simulink model "kinovaMicoSimscapeModel"  (R2021b)
(part 42 of 50)

Y6_20_4=(3*dq2*dqr3*sin(2*q6))/128 + (3*dq3*dqr2*sin(2*q6))/128 - (3*dq3*dqr3*sin(2*q6))/128 + (3*dq2*dqr3*cos(2*q6)*sin(q5))/16 + (3*dq2*dqr3*sin(2*q6)*cos(q5))/32 - (3*dq3*dqr3*cos(2*q6)*sin(q5))/16 - (3*dq3*dqr3*sin(2*q6)*cos(q5))/32 + (3^(1/2)*dq4*dqr3*sin(q4))/8 + (27*dq2*dqr3*cos(2*q4)*sin(2*q6))/128 + (27*dq3*dqr2*cos(2*q4)*sin(2*q6))/128 - (15*dq2*dqr3*cos(2*q5)*sin(2*q6))/128 - (3*dq2*dqr3*cos(2*q6)*sin(2*q5))/32 - (15*dq3*dqr2*cos(2*q5)*sin(2*q6))/128 - (27*dq3*dqr3*cos(2*q4)*sin(2*q6))/128 + (15*dq3*dqr3*cos(2*q5)*sin(2*q6))/128 + (3*dq3*dqr3*cos(2*q6)*sin(2*q5))/32 - (dq1*dqr3*cos(q2)*sin(q3))/8 + (dq1*dqr3*cos(q3)*sin(q2))/8 - (3^(1/2)*dq4*dqr3*cos(q4)*sin(q5))/4 - (3^(1/2)*dq4*dqr3*cos(q5)*sin(q4))/8 - (3^(1/2)*dq5*dqr3*cos(q4)*sin(q5))/8 - (3^(1/2)*dq5*dqr3*cos(q5)*sin(q4))/4 + (3*dq2*dqr3*cos(2*q4)*cos(2*q6)*sin(q5))/16 + (3*dq2*dqr3*cos(2*q4)*sin(2*q6)*cos(q5))/32 + (3*dq2*dqr3*cos(2*q6)*sin(2*q4)*cos(q5))/8 - (3*dq3*dqr3*cos(2*q4)*cos(2*q6)*sin(q5))/16 - (3*dq3*dqr3*cos(2*q4)*sin(2*q6)*cos(q5))/32 - (3*dq3*dqr3*cos(2*q6)*sin(2*q4)*cos(q5))/8 - (3*dq2*dqr3*sin(2*q4)*sin(2*q6)*sin(q5))/16 + (3*dq3*dqr3*sin(2*q4)*sin(2*q6)*sin(q5))/16 + (9*3^(1/2)*dq4*dqr3*sin(2*q6)*cos(q4))/64 + (3*3^(1/2)*dq5*dqr3*sin(2*q6)*cos(q4))/16 - (3*dq1*dqr3*cos(q2)*cos(q5)*sin(q3))/8 + (3*dq1*dqr3*cos(q3)*cos(q5)*sin(q2))/8 + (25*dq2*dqr3*cos(2*q4)*cos(2*q5)*sin(2*q6))/128 + (5*dq2*dqr3*cos(2*q4)*cos(2*q6)*sin(2*q5))/32 + (dq2*dqr3*cos(2*q5)*cos(2*q6)*sin(2*q4))/8 + (25*dq3*dqr2*cos(2*q4)*cos(2*q5)*sin(2*q6))/128 - (25*dq3*dqr3*cos(2*q4)*cos(2*q5)*sin(2*q6))/128 - (5*dq3*dqr3*cos(2*q4)*cos(2*q6)*sin(2*q5))/32 - (dq3*dqr3*cos(2*q5)*cos(2*q6)*sin(2*q4))/8 - (5*dq2*dqr3*sin(2*q4)*sin(2*q5)*sin(2*q6))/32 + (5*dq3*dqr3*sin(2*q4)*sin(2*q5)*sin(2*q6))/32 + (3*dq1*dqr4*cos(2*q6)*sin(q2)*sin(q3)*sin(q5))/8 + (3*dq1*dqr4*sin(2*q6)*cos(q5)*sin(q2)*sin(q3))/16 - (3^(1/2)*dq1*dqr3*cos(q2)*cos(q3)*sin(q4))/8 - (3^(1/2)*dq1*dqr3*sin(q2)*sin(q3)*sin(q4))/8 - (27*dq1*dqr3*sin(2*q4)*sin(2*q6)*cos(q2)*sin(q3))/128 + (27*dq1*dqr3*sin(2*q4)*sin(2*q6)*cos(q3)*sin(q2))/128 - (3*dq1*dqr4*cos(2*q6)*sin(2*q5)*sin(q2)*sin(q3))/16 - (3^(1/2)*dq4*dqr3*cos(2*q6)*cos(q4)*sin(q5))/8 + (3^(1/2)*dq4*dqr3*cos(2*q6)*cos(q5)*sin(q4))/8 - (3^(1/2)*dq4*dqr3*sin(2*q6)*cos(q4)*cos(q5))/16 + (3^(1/2)*dq5*dqr3*cos(2*q6)*cos(q4)*sin(q5))/8 + (3^(1/2)*dq5*dqr3*cos(2*q6)*cos(q5)*sin(q4))/4 + (3^(1/2)*dq5*dqr3*sin(2*q6)*cos(q4)*cos(q5))/16 - (3^(1/2)*dq4*dqr3*sin(2*q6)*sin(q4)*sin(q5))/16 - (3^(1/2)*dq5*dqr3*sin(2*q6)*sin(q4)*sin(q5))/8 - (3^(1/2)*dq4*dqr3*cos(2*q5)*cos(2*q6)*sin(q4))/8 - (5*3^(1/2)*dq4*dqr3*cos(2*q5)*sin(2*q6)*cos(q4))/64 - (3^(1/2)*dq4*dqr3*cos(2*q6)*sin(2*q5)*cos(q4))/16 + (5*3^(1/2)*dq4*dqr3*sin(2*q5)*sin(2*q6)*sin(q4))/32 + (3^(1/2)*dq1*dqr3*cos(q4)*sin(q2)*sin(q3)*sin(q5))/4 + (3^(1/2)*dq1*dqr3*cos(q5)*sin(q2)*sin(q3)*sin(q4))/8 + (3*dq1*dqr3*cos(2*q4)*cos(2*q6)*cos(q2)*cos(q5)*sin(q3))/8 - (3*dq1*dqr3*cos(2*q4)*cos(2*q6)*cos(q3)*cos(q5)*sin(q2))/8 - (3*dq1*dqr3*cos(2*q4)*sin(2*q6)*cos(q2)*sin(q3)*sin(q5))/16 + (3*dq1*dqr3*cos(2*q4)*sin(2*q6)*cos(q3)*sin(q2)*sin(q5))/16 - (3*dq1*dqr3*cos(2*q6)*sin(2*q4)*cos(q2)*sin(q3)*sin(q5))/16 + (3*dq1*dqr3*cos(2*q6)*sin(2*q4)*cos(q3)*sin(q2)*sin(q5))/16 - (3*dq1*dqr3*sin(2*q4)*sin(2*q6)*cos(q2)*cos(q5)*sin(q3))/32 + (3*dq1*dqr3*sin(2*q4)*sin(2*q6)*cos(q3)*cos(q5)*sin(q2))/32 + (9*3^(1/2)*dq1*dqr3*sin(2*q6)*cos(q2)*cos(q3)*cos(q4))/64 + (9*3^(1/2)*dq1*dqr3*sin(2*q6)*cos(q4)*sin(q2)*sin(q3))/64 + (dq1*dqr3*cos(2*q4)*cos(2*q5)*cos(2*q6)*cos(q2)*sin(q3))/8 - (dq1*dqr3*cos(2*q4)*cos(2*q5)*cos(2*q6)*cos(q3)*sin(q2))/8 - (5*dq1*dqr3*cos(2*q4)*sin(2*q5)*sin(2*q6)*cos(q2)*sin(q3))/32 + (5*dq1*dqr3*cos(2*q4)*sin(2*q5)*sin(2*q6)*cos(q3)*sin(q2))/32 - (25*dq1*dqr3*cos(2*q5)*sin(2*q4)*sin(2*q6)*cos(q2)*sin(q3))/128 + (25*dq1*dqr3*cos(2*q5)*sin(2*q4)*sin(2*q6)*cos(q3)*sin(q2))/128 - (5*dq1*dqr3*cos(2*q6)*sin(2*q4)*sin(2*q5)*cos(q2)*sin(q3))/32 + (5*dq1*dqr3*cos(2*q6)*sin(2*q4)*sin(2*q5)*cos(q3)*sin(q2))/32 + (3^(1/2)*dq1*dqr3*cos(q2)*cos(q3)*cos(q4)*sin(q5))/4 + (3^(1/2)*dq1*dqr3*cos(q2)*cos(q3)*cos(q5)*sin(q4))/8 - (3^(1/2)*dq1*dqr3*cos(2*q6)*cos(q2)*cos(q3)*cos(q4)*sin(q5))/8 + (3^(1/2)*dq1*dqr3*cos(2*q6)*cos(q2)*cos(q3)*cos(q5)*sin(q4))/8 - (3^(1/2)*dq1*dqr3*sin(2*q6)*cos(q2)*cos(q3)*cos(q4)*cos(q5))/16 - (3^(1/2)*dq1*dqr3*cos(2*q6)*cos(q4)*sin(q2)*sin(q3)*sin(q5))/8 + (3^(1/2)*dq1*dqr3*cos(2*q6)*cos(q5)*sin(q2)*sin(q3)*sin(q4))/8 - (3^(1/2)*dq1*dqr3*sin(2*q6)*cos(q2)*cos(q3)*sin(q4)*sin(q5))/16 - (3^(1/2)*dq1*dqr3*sin(2*q6)*cos(q4)*cos(q5)*sin(q2)*sin(q3))/16 - (3^(1/2)*dq1*dqr3*sin(2*q6)*sin(q2)*sin(q3)*sin(q4)*sin(q5))/16 - (3^(1/2)*dq1*dqr3*cos(2*q5)*cos(2*q6)*cos(q2)*cos(q3)*sin(q4))/8 - (5*3^(1/2)*dq1*dqr3*cos(2*q5)*sin(2*q6)*cos(q2)*cos(q3)*cos(q4))/64 - (3^(1/2)*dq1*dqr3*cos(2*q6)*sin(2*q5)*cos(q2)*cos(q3)*cos(q4))/16 - (3^(1/2)*dq1*dqr3*cos(2*q5)*cos(2*q6)*sin(q2)*sin(q3)*sin(q4))/8 - (5*3^(1/2)*dq1*dqr3*cos(2*q5)*sin(2*q6)*cos(q4)*sin(q2)*sin(q3))/64 - (3^(1/2)*dq1*dqr3*cos(2*q6)*sin(2*q5)*cos(q4)*sin(q2)*sin(q3))/16 + (5*3^(1/2)*dq1*dqr3*sin(2*q5)*sin(2*q6)*cos(q2)*cos(q3)*sin(q4))/32 + (5*3^(1/2)*dq1*dqr3*sin(2*q5)*sin(2*q6)*sin(q2)*sin(q3)*sin(q4))/32;
Y6_20_5=(3*dq4*dqr4*sin(2*q6))/64 - (3*dq5*dqr4*sin(q5))/8 - (3*dq4*dqr5*sin(q5))/8 - (3*dq5*dqr4*sin(2*q6))/16 + (3*dq4*dqr4*cos(2*q6)*sin(q5))/8 + (3*dq4*dqr4*sin(2*q6)*cos(q5))/16 + (3*dq4*dqr5*cos(2*q6)*sin(q5))/8 + (3*dq5*dqr4*cos(2*q6)*sin(q5))/8 + (3*dq5*dqr4*sin(2*q6)*cos(q5))/16 - (3^(1/2)*dq2*dqr4*sin(q4))/8 + (3^(1/2)*dq3*dqr4*sin(q4))/8 - (15*dq4*dqr4*cos(2*q5)*sin(2*q6))/64 - (3*dq4*dqr4*cos(2*q6)*sin(2*q5))/16 + (3*dq1*dqr4*sin(2*q6)*cos(q2)*cos(q3))/64 - (3*dq1*dqr5*sin(2*q6)*cos(q2)*cos(q3))/16 + (3*dq1*dqr4*sin(2*q6)*sin(q2)*sin(q3))/64 - (3*dq1*dqr5*sin(2*q6)*sin(q2)*sin(q3))/16 + (3^(1/2)*dq2*dqr4*cos(q4)*sin(q5))/4 + (3^(1/2)*dq2*dqr4*cos(q5)*sin(q4))/8 + (3^(1/2)*dq2*dqr5*cos(q4)*sin(q5))/8 + (3^(1/2)*dq2*dqr5*cos(q5)*sin(q4))/4 - (3^(1/2)*dq3*dqr4*cos(q4)*sin(q5))/4 - (3^(1/2)*dq3*dqr4*cos(q5)*sin(q4))/8 - (3^(1/2)*dq3*dqr5*cos(q4)*sin(q5))/8 - (3^(1/2)*dq3*dqr5*cos(q5)*sin(q4))/4 - (9*3^(1/2)*dq2*dqr4*sin(2*q6)*cos(q4))/64 + (9*3^(1/2)*dq3*dqr4*sin(2*q6)*cos(q4))/64 - (3*dq1*dqr5*cos(q2)*cos(q3)*sin(q5))/8 - (3*dq1*dqr5*sin(q2)*sin(q3)*sin(q5))/8 + (3*dq1*dqr5*cos(2*q6)*sin(q2)*sin(q3)*sin(q5))/8 + (3*dq1*dqr5*sin(2*q6)*cos(q5)*sin(q2)*sin(q3))/16 - (3^(1/2)*dq1*dqr4*cos(q2)*cos(q4)*sin(q3))/8 + (3^(1/2)*dq1*dqr4*cos(q3)*cos(q4)*sin(q2))/8 - (15*dq1*dqr4*cos(2*q5)*sin(2*q6)*cos(q2)*cos(q3))/64 - (3*dq1*dqr4*cos(2*q6)*sin(2*q5)*cos(q2)*cos(q3))/16 - (15*dq1*dqr4*cos(2*q5)*sin(2*q6)*sin(q2)*sin(q3))/64 + (3^(1/2)*dq2*dqr4*cos(2*q6)*cos(q4)*sin(q5))/8 - (3^(1/2)*dq2*dqr4*cos(2*q6)*cos(q5)*sin(q4))/8 + (3^(1/2)*dq2*dqr4*sin(2*q6)*cos(q4)*cos(q5))/16 - (3^(1/2)*dq2*dqr5*cos(2*q6)*cos(q4)*sin(q5))/8 - (3^(1/2)*dq2*dqr5*cos(2*q6)*cos(q5)*sin(q4))/4 - (3^(1/2)*dq2*dqr5*sin(2*q6)*cos(q4)*cos(q5))/16 - (3^(1/2)*dq3*dqr4*cos(2*q6)*cos(q4)*sin(q5))/8 + (3^(1/2)*dq3*dqr4*cos(2*q6)*cos(q5)*sin(q4))/8 - (3^(1/2)*dq3*dqr4*sin(2*q6)*cos(q4)*cos(q5))/16 + (3^(1/2)*dq3*dqr5*cos(2*q6)*cos(q4)*sin(q5))/8 + (3^(1/2)*dq3*dqr5*cos(2*q6)*cos(q5)*sin(q4))/4 + (3^(1/2)*dq3*dqr5*sin(2*q6)*cos(q4)*cos(q5))/16 + (3^(1/2)*dq2*dqr4*sin(2*q6)*sin(q4)*sin(q5))/16 + (3^(1/2)*dq2*dqr5*sin(2*q6)*sin(q4)*sin(q5))/8 - (3^(1/2)*dq3*dqr4*sin(2*q6)*sin(q4)*sin(q5))/16 - (3^(1/2)*dq3*dqr5*sin(2*q6)*sin(q4)*sin(q5))/8 + (3^(1/2)*dq2*dqr4*cos(2*q5)*cos(2*q6)*sin(q4))/8 + (5*3^(1/2)*dq2*dqr4*cos(2*q5)*sin(2*q6)*cos(q4))/64 + (3^(1/2)*dq2*dqr4*cos(2*q6)*sin(2*q5)*cos(q4))/16 - (3^(1/2)*dq3*dqr4*cos(2*q5)*cos(2*q6)*sin(q4))/8 - (5*3^(1/2)*dq3*dqr4*cos(2*q5)*sin(2*q6)*cos(q4))/64 - (3^(1/2)*dq3*dqr4*cos(2*q6)*sin(2*q5)*cos(q4))/16 + (3*dq1*dqr4*cos(2*q6)*cos(q2)*cos(q3)*sin(q5))/8 + (3*dq1*dqr4*sin(2*q6)*cos(q2)*cos(q3)*cos(q5))/16 + (3*dq1*dqr5*cos(2*q6)*cos(q2)*cos(q3)*sin(q5))/8 + (3*dq1*dqr5*sin(2*q6)*cos(q2)*cos(q3)*cos(q5))/16 - (5*3^(1/2)*dq2*dqr4*sin(2*q5)*sin(2*q6)*sin(q4))/32 + (5*3^(1/2)*dq3*dqr4*sin(2*q5)*sin(2*q6)*sin(q4))/32 - (3^(1/2)*dq1*dqr4*cos(q2)*sin(q3)*sin(q4)*sin(q5))/4 + (3^(1/2)*dq1*dqr4*cos(q3)*sin(q2)*sin(q4)*sin(q5))/4 - (3^(1/2)*dq1*dqr5*cos(q2)*sin(q3)*sin(q4)*sin(q5))/8 + (3^(1/2)*dq1*dqr5*cos(q3)*sin(q2)*sin(q4)*sin(q5))/8 + (9*3^(1/2)*dq1*dqr4*sin(2*q6)*cos(q2)*sin(q3)*sin(q4))/64 - (9*3^(1/2)*dq1*dqr4*sin(2*q6)*cos(q3)*sin(q2)*sin(q4))/64 + (3*3^(1/2)*dq1*dqr5*sin(2*q6)*cos(q2)*sin(q3)*sin(q4))/16 - (3*3^(1/2)*dq1*dqr5*sin(2*q6)*cos(q3)*sin(q2)*sin(q4))/16 + (3^(1/2)*dq1*dqr4*cos(q2)*cos(q4)*cos(q5)*sin(q3))/8 - (3^(1/2)*dq1*dqr4*cos(q3)*cos(q4)*cos(q5)*sin(q2))/8 + (3^(1/2)*dq1*dqr5*cos(q2)*cos(q4)*cos(q5)*sin(q3))/4 - (3^(1/2)*dq1*dqr5*cos(q3)*cos(q4)*cos(q5)*sin(q2))/4 - (3^(1/2)*dq1*dqr4*cos(2*q6)*cos(q2)*cos(q4)*cos(q5)*sin(q3))/8 + (3^(1/2)*dq1*dqr4*cos(2*q6)*cos(q3)*cos(q4)*cos(q5)*sin(q2))/8 - (3^(1/2)*dq1*dqr5*cos(2*q6)*cos(q2)*cos(q4)*cos(q5)*sin(q3))/4 + (3^(1/2)*dq1*dqr5*cos(2*q6)*cos(q3)*cos(q4)*cos(q5)*sin(q2))/4 - (3^(1/2)*dq1*dqr4*cos(2*q6)*cos(q2)*sin(q3)*sin(q4)*sin(q5))/8 + (3^(1/2)*dq1*dqr4*cos(2*q6)*cos(q3)*sin(q2)*sin(q4)*sin(q5))/8 + (3^(1/2)*dq1*dqr4*sin(2*q6)*cos(q2)*cos(q4)*sin(q3)*sin(q5))/16 - (3^(1/2)*dq1*dqr4*sin(2*q6)*cos(q2)*cos(q5)*sin(q3)*sin(q4))/16 - (3^(1/2)*dq1*dqr4*sin(2*q6)*cos(q3)*cos(q4)*sin(q2)*sin(q5))/16 + (3^(1/2)*dq1*dqr4*sin(2*q6)*cos(q3)*cos(q5)*sin(q2)*sin(q4))/16 + (3^(1/2)*dq1*dqr5*cos(2*q6)*cos(q2)*sin(q3)*sin(q4)*sin(q5))/8 - (3^(1/2)*dq1*dqr5*cos(2*q6)*cos(q3)*sin(q2)*sin(q4)*sin(q5))/8 + (3^(1/2)*dq1*dqr5*sin(2*q6)*cos(q2)*cos(q4)*sin(q3)*sin(q5))/8 + (3^(1/2)*dq1*dqr5*sin(2*q6)*cos(q2)*cos(q5)*sin(q3)*sin(q4))/16 - (3^(1/2)*dq1*dqr5*sin(2*q6)*cos(q3)*cos(q4)*sin(q2)*sin(q5))/8 - (3^(1/2)*dq1*dqr5*sin(2*q6)*cos(q3)*cos(q5)*sin(q2)*sin(q4))/16 + (3^(1/2)*dq1*dqr4*cos(2*q5)*cos(2*q6)*cos(q2)*cos(q4)*sin(q3))/8 - (3^(1/2)*dq1*dqr4*cos(2*q5)*cos(2*q6)*cos(q3)*cos(q4)*sin(q2))/8 - (5*3^(1/2)*dq1*dqr4*cos(2*q5)*sin(2*q6)*cos(q2)*sin(q3)*sin(q4))/64 + (5*3^(1/2)*dq1*dqr4*cos(2*q5)*sin(2*q6)*cos(q3)*sin(q2)*sin(q4))/64 - (3^(1/2)*dq1*dqr4*cos(2*q6)*sin(2*q5)*cos(q2)*sin(q3)*sin(q4))/16 + (3^(1/2)*dq1*dqr4*cos(2*q6)*sin(2*q5)*cos(q3)*sin(q2)*sin(q4))/16 - (5*3^(1/2)*dq1*dqr4*sin(2*q5)*sin(2*q6)*cos(q2)*cos(q4)*sin(q3))/32 + (5*3^(1/2)*dq1*dqr4*sin(2*q5)*sin(2*q6)*cos(q3)*cos(q4)*sin(q2))/32;
Y6_20_6=ddqr4/4 + ddqr5/2 + ddqr6 + (3*ddqr4*cos(q5))/4 + (ddqr1*cos(q2 - q3))/4 - (3*dq4*dqr5*sin(2*q6))/16 - (3*dq5*dqr5*sin(2*q6))/8 + (3*ddqr1*cos(q2 - q3)*cos(q5))/4 + (3^(1/2)*ddqr2*cos(q4))/4 - (3^(1/2)*ddqr3*cos(q4))/4 + (3*dq4*dqr5*sin(2*q6)*cos(q5))/16 - (3^(1/2)*ddqr2*cos(q4)*cos(q5))/4 + (3^(1/2)*ddqr3*cos(q4)*cos(q5))/4 + (3^(1/2)*ddqr2*sin(q4)*sin(q5))/2 - (3^(1/2)*ddqr3*sin(q4)*sin(q5))/2 - (3*3^(1/2)*dq2*dqr5*sin(2*q6)*cos(q4))/16 + (3*3^(1/2)*dq3*dqr5*sin(2*q6)*cos(q4))/16;
Y6_25_1=(3*cos(q3 - q2 + q4)*sin(q6))/8 - (3*cos(q2 - q3 + q4)*sin(q6))/8 + (3^(1/2)*cos(q2 - q3)*sin(q6))/4 - (3^(1/2)*cos(q2 - q3)*cos(q5)*sin(q6))/4 - (3^(1/2)*cos(q2 - q3)*cos(q6)*sin(q5))/2 + cos(q2)*cos(q4)*cos(q5)*cos(q6)*sin(q3) - cos(q3)*cos(q4)*cos(q5)*cos(q6)*sin(q2) - (cos(q2)*cos(q4)*sin(q3)*sin(q5)*sin(q6))/2 - (cos(q2)*cos(q5)*sin(q3)*sin(q4)*sin(q6))/4 - (cos(q2)*cos(q6)*sin(q3)*sin(q4)*sin(q5))/2 + (cos(q3)*cos(q4)*sin(q2)*sin(q5)*sin(q6))/2 + (cos(q3)*cos(q5)*sin(q2)*sin(q4)*sin(q6))/4 + (cos(q3)*cos(q6)*sin(q2)*sin(q4)*sin(q5))/2;

%% Here are all the sums of the terms
Y1_1=Y1_1_1; 
Y1_2=Y1_2_1; 
Y1_3=Y1_3_1; 
Y1_4=Y1_4_1 + Y1_4_2; 
Y1_5=Y1_5_1 + Y1_5_2 + Y1_5_3 + Y1_5_4 + Y1_5_5 + Y1_5_6 + Y1_5_7 + Y1_5_8 + Y1_5_9; 
Y1_6=Y1_6_1; 
Y1_7=Y1_7_1; 
Y1_8=Y1_8_1; 
Y1_9=Y1_9_1 + Y1_9_2 + Y1_9_3 + Y1_9_4 + Y1_9_5; 
Y1_10=Y1_10_1 + Y1_10_2 + Y1_10_3 + Y1_10_4 + Y1_10_5 + Y1_10_6 + Y1_10_7 + Y1_10_8 + Y1_10_9 + Y1_10_10 + Y1_10_11 + Y1_10_12 + Y1_10_13 + Y1_10_14 + Y1_10_15 + Y1_10_16 + Y1_10_17 + Y1_10_18 + Y1_10_19 + Y1_10_20 + Y1_10_21 + Y1_10_22; 
Y1_15=Y1_15_1; 
Y1_16=Y1_16_1; 
Y1_17=Y1_17_1; 
Y1_18=Y1_18_1; 
Y1_19=Y1_19_1 + Y1_19_2 + Y1_19_3 + Y1_19_4; 
Y1_20=Y1_20_1 + Y1_20_2 + Y1_20_3 + Y1_20_4 + Y1_20_5 + Y1_20_6 + Y1_20_7 + Y1_20_8 + Y1_20_9 + Y1_20_10 + Y1_20_11 + Y1_20_12 + Y1_20_13 + Y1_20_14 + Y1_20_15 + Y1_20_16 + Y1_20_17 + Y1_20_18 + Y1_20_19 + Y1_20_20 + Y1_20_21; 
Y2_2=Y2_2_1; 
Y2_3=Y2_3_1; 
Y2_4=Y2_4_1; 
Y2_5=Y2_5_1 + Y2_5_2 + Y2_5_3 + Y2_5_4; 
Y2_6=Y2_6_1; 
Y2_7=Y2_7_1; 
Y2_8=Y2_8_1; 
Y2_9=Y2_9_1 + Y2_9_2; 
Y2_10=Y2_10_1 + Y2_10_2 + Y2_10_3 + Y2_10_4 + Y2_10_5 + Y2_10_6 + Y2_10_7 + Y2_10_8 + Y2_10_9 + Y2_10_10; 
Y2_11=Y2_11_1; 
Y2_12=Y2_12_1; 
Y2_13=Y2_13_1; 
Y2_14=Y2_14_1; 
Y2_16=Y2_16_1; 
Y2_17=Y2_17_1; 
Y2_18=Y2_18_1; 
Y2_19=Y2_19_1 + Y2_19_2; 
Y2_20=Y2_20_1 + Y2_20_2 + Y2_20_3 + Y2_20_4 + Y2_20_5 + Y2_20_6 + Y2_20_7 + Y2_20_8 + Y2_20_9 + Y2_20_10; 
Y2_21=Y2_21_1; 
Y2_22=Y2_22_1; 
Y2_23=Y2_23_1; 
Y2_24=Y2_24_1; 
Y2_25=Y2_25_1; 
Y3_3=Y3_3_1; 
Y3_4=Y3_4_1; 
Y3_5=Y3_5_1 + Y3_5_2 + Y3_5_3; 
Y3_7=Y3_7_1; 
Y3_8=Y3_8_1; 
Y3_9=Y3_9_1 + Y3_9_2; 
Y3_10=Y3_10_1 + Y3_10_2 + Y3_10_3 + Y3_10_4 + Y3_10_5 + Y3_10_6 + Y3_10_7; 
Y3_12=Y3_12_1; 
Y3_13=Y3_13_1; 
Y3_14=Y3_14_1; 
Y3_17=Y3_17_1; 
Y3_18=Y3_18_1; 
Y3_19=Y3_19_1 + Y3_19_2; 
Y3_20=Y3_20_1 + Y3_20_2 + Y3_20_3 + Y3_20_4 + Y3_20_5 + Y3_20_6 + Y3_20_7 + Y3_20_8 + Y3_20_9; 
Y3_22=Y3_22_1; 
Y3_23=Y3_23_1; 
Y3_24=Y3_24_1; 
Y3_25=Y3_25_1; 
Y4_4=Y4_4_1; 
Y4_5=Y4_5_1 + Y4_5_2 + Y4_5_3; 
Y4_8=Y4_8_1; 
Y4_9=Y4_9_1 + Y4_9_2; 
Y4_10=Y4_10_1 + Y4_10_2 + Y4_10_3 + Y4_10_4 + Y4_10_5 + Y4_10_6 + Y4_10_7; 
Y4_13=Y4_13_1; 
Y4_14=Y4_14_1; 
Y4_18=Y4_18_1; 
Y4_19=Y4_19_1 + Y4_19_2; 
Y4_20=Y4_20_1 + Y4_20_2 + Y4_20_3 + Y4_20_4 + Y4_20_5 + Y4_20_6 + Y4_20_7 + Y4_20_8 + Y4_20_9; 
Y4_23=Y4_23_1; 
Y4_24=Y4_24_1; 
Y4_25=Y4_25_1; 
Y5_5=Y5_5_1 + Y5_5_2 + Y5_5_3; 
Y5_9=Y5_9_1 + Y5_9_2; 
Y5_10=Y5_10_1 + Y5_10_2 + Y5_10_3 + Y5_10_4 + Y5_10_5 + Y5_10_6; 
Y5_14=Y5_14_1; 
Y5_19=Y5_19_1 + Y5_19_2; 
Y5_20=Y5_20_1 + Y5_20_2 + Y5_20_3 + Y5_20_4 + Y5_20_5 + Y5_20_6 + Y5_20_7; 
Y5_24=Y5_24_1; 
Y5_25=Y5_25_1; 
Y6_10=Y6_10_1 + Y6_10_2 + Y6_10_3 + Y6_10_4 + Y6_10_5 + Y6_10_6; 
Y6_20=Y6_20_1 + Y6_20_2 + Y6_20_3 + Y6_20_4 + Y6_20_5 + Y6_20_6; 
Y6_25=Y6_25_1; 

%% Here is the entire regressor matrix
Y=[Y1_1, Y1_2, Y1_3, Y1_4, Y1_5, Y1_6, Y1_7, Y1_8, Y1_9, Y1_10,     0,     0,     0,     0, Y1_15, Y1_16, Y1_17, Y1_18, Y1_19, Y1_20,     0,     0,     0,     0,     0;
   0, Y2_2, Y2_3, Y2_4, Y2_5, Y2_6, Y2_7, Y2_8, Y2_9, Y2_10, Y2_11, Y2_12, Y2_13, Y2_14,     0, Y2_16, Y2_17, Y2_18, Y2_19, Y2_20, Y2_21, Y2_22, Y2_23, Y2_24, Y2_25;
   0,    0, Y3_3, Y3_4, Y3_5,    0, Y3_7, Y3_8, Y3_9, Y3_10,     0, Y3_12, Y3_13, Y3_14,     0,     0, Y3_17, Y3_18, Y3_19, Y3_20,     0, Y3_22, Y3_23, Y3_24, Y3_25;
   0,    0,    0, Y4_4, Y4_5,    0,    0, Y4_8, Y4_9, Y4_10,     0,     0, Y4_13, Y4_14,     0,     0,     0, Y4_18, Y4_19, Y4_20,     0,     0, Y4_23, Y4_24, Y4_25;
   0,    0,    0,    0, Y5_5,    0,    0,    0, Y5_9, Y5_10,     0,     0,     0, Y5_14,     0,     0,     0,     0, Y5_19, Y5_20,     0,     0,     0, Y5_24, Y5_25;
   0,    0,    0,    0,    0,    0,    0,    0,    0, Y6_10,     0,     0,     0,     0,     0,     0,     0,     0,     0, Y6_20,     0,     0,     0,     0, Y6_25];
